simulink model "allmodes"  (Simulink 7.4)
settings: Solver=ode23tb  StartTime=0.0  StopTime=inf  MaxStep=1e-4  RelTol=1e-4
undefined symbols (not defined in the file): Ion, Lithium
libraries: powerlib x185, electricdrivelib x21, powerlib_extras x19, simulink x5
(part 6 of 7)

== system allmodes/battery controller /v16/Subsystem ==
  In1 : Inport
  Enable : EnablePort
  Constant2 : Constant  Value=0  OutDataType=fixdt(1, 16)  OutScaling=2^0
  Data Type Conversion2 : DataTypeConversion  OutDataType=fixdt(1, 16)  OutScaling=2^0
  Data Type Conversion3 : DataTypeConversion  OutDataType=fixdt(1, 16)  OutScaling=2^0
  Gain1 : Gain  Gain=-1  ParameterDataType=fixdt(1, 16)  ParameterScaling=2^0  OutDataType=fixdt(1, 16)  OutScaling=2^0
  Relational Operator2 : RelationalOperator  Operator=>  LogicOutDataTypeMode=boolean  LogicDataType=fixdt(0, 8)  OutDataTypeStr=boolean
  Relational Operator3 : RelationalOperator  Operator=>  LogicOutDataTypeMode=boolean  LogicDataType=fixdt(0, 8)  OutDataTypeStr=boolean
  Switch1 : Switch  OutDataType=fixdt(1, 16)  OutScaling=2^0
  Switch2 : Switch  Criteria=u2 > Threshold  OutDataType=fixdt(1, 16)  OutScaling=2^0
  sawtooth generator : Subsystem  mask{fsw=5e3, vc=1}
      mask prompts: fsw "switching frequency"; vc "magnitude"
  Out1 : Outport
  Out2 : Outport  Port=2
  wires:
  Switch1/1 -> Out2/1
  Switch2/1 -> Out1/1
  In1/1 -> Relational Operator2/1, Switch2/2, Switch1/2, Gain1/1
  Relational Operator3/1 -> Data Type Conversion2/1
  Relational Operator2/1 -> Data Type Conversion3/1
  Data Type Conversion3/1 -> Switch2/1
  Constant2/1 -> Switch2/3, Switch1/1
  Data Type Conversion2/1 -> Switch1/3
  sawtooth generator/1(saw) -> Relational Operator3/2, Relational Operator2/2
  Gain1/1 -> Relational Operator3/1

== system allmodes/battery controller /v16/Subsystem1 ==
  In1 : Inport
  Integrator : Integrator
  ain9 : Gain  Gain=5  ParameterDataType=fixdt(1, 16)  ParameterScaling=2^0  OutDataType=fixdt(1, 16)  OutScaling=2^0
  Out1 : Outport
  wires:
  In1/1 -> ain9/1
  Integrator/1 -> Out1/1
  ain9/1 -> Integrator/1

== system allmodes/battery controller /v16/Subsystem2 ==
  In1 : Inport
  Integrator : Integrator
  ain9 : Gain  Gain=5  ParameterDataType=fixdt(1, 16)  ParameterScaling=2^0  OutDataType=fixdt(1, 16)  OutScaling=2^0
  Out1 : Outport
  wires:
  ain9/1 -> Integrator/1
  Integrator/1 -> Out1/1
  In1/1 -> ain9/1

== system allmodes/battery controller /v16/Subsystem3 ==
  In1 : Inport
  Integrator : Integrator
  ain9 : Gain  Gain=5  ParameterDataType=fixdt(1, 16)  ParameterScaling=2^0  OutDataType=fixdt(1, 16)  OutScaling=2^0
  Out1 : Outport
  wires:
  In1/1 -> ain9/1
  Integrator/1 -> Out1/1
  ain9/1 -> Integrator/1

== system allmodes/battery controller /v17/Subsystem ==
  In1 : Inport
  Enable : EnablePort
  Constant2 : Constant  Value=0  OutDataType=fixdt(1, 16)  OutScaling=2^0
  Data Type Conversion2 : DataTypeConversion  OutDataType=fixdt(1, 16)  OutScaling=2^0
  Data Type Conversion3 : DataTypeConversion  OutDataType=fixdt(1, 16)  OutScaling=2^0
  Gain1 : Gain  Gain=-1  ParameterDataType=fixdt(1, 16)  ParameterScaling=2^0  OutDataType=fixdt(1, 16)  OutScaling=2^0
  Relational Operator2 : RelationalOperator  Operator=>  LogicOutDataTypeMode=boolean  LogicDataType=fixdt(0, 8)  OutDataTypeStr=boolean
  Relational Operator3 : RelationalOperator  Operator=>  LogicOutDataTypeMode=boolean  LogicDataType=fixdt(0, 8)  OutDataTypeStr=boolean
  Switch1 : Switch  OutDataType=fixdt(1, 16)  OutScaling=2^0
  Switch2 : Switch  Criteria=u2 > Threshold  OutDataType=fixdt(1, 16)  OutScaling=2^0
  sawtooth generator : Subsystem  mask{fsw=5e3, vc=1}
      mask prompts: fsw "switching frequency"; vc "magnitude"
  Out1 : Outport
  Out2 : Outport  Port=2
  wires:
  Switch1/1 -> Out2/1
  Switch2/1 -> Out1/1
  In1/1 -> Relational Operator2/1, Switch2/2, Switch1/2, Gain1/1
  Relational Operator3/1 -> Data Type Conversion2/1
  Relational Operator2/1 -> Data Type Conversion3/1
  Data Type Conversion3/1 -> Switch2/1
  Constant2/1 -> Switch2/3, Switch1/1
  Data Type Conversion2/1 -> Switch1/3
  sawtooth generator/1(saw) -> Relational Operator3/2, Relational Operator2/2
  Gain1/1 -> Relational Operator3/1

== system allmodes/battery controller /v17/Subsystem1 ==
  In1 : Inport
  Integrator : Integrator
  ain9 : Gain  Gain=5  ParameterDataType=fixdt(1, 16)  ParameterScaling=2^0  OutDataType=fixdt(1, 16)  OutScaling=2^0
  Out1 : Outport
  wires:
  In1/1 -> ain9/1
  Integrator/1 -> Out1/1
  ain9/1 -> Integrator/1

== system allmodes/battery controller /v17/Subsystem2 ==
  In1 : Inport
  Integrator : Integrator
  ain9 : Gain  Gain=5  ParameterDataType=fixdt(1, 16)  ParameterScaling=2^0  OutDataType=fixdt(1, 16)  OutScaling=2^0
  Out1 : Outport
  wires:
  ain9/1 -> Integrator/1
  Integrator/1 -> Out1/1
  In1/1 -> ain9/1

== system allmodes/battery controller /v17/Subsystem3 ==
  In1 : Inport
  Integrator : Integrator
  ain9 : Gain  Gain=5  ParameterDataType=fixdt(1, 16)  ParameterScaling=2^0  OutDataType=fixdt(1, 16)  OutScaling=2^0
  Out1 : Outport
  wires:
  In1/1 -> ain9/1
  Integrator/1 -> Out1/1
  ain9/1 -> Integrator/1

== system allmodes/battery controller /v18/Subsystem ==
  In1 : Inport
  Enable : EnablePort
  Constant2 : Constant  Value=0  OutDataType=fixdt(1, 16)  OutScaling=2^0
  Data Type Conversion2 : DataTypeConversion  OutDataType=fixdt(1, 16)  OutScaling=2^0
  Data Type Conversion3 : DataTypeConversion  OutDataType=fixdt(1, 16)  OutScaling=2^0
  Gain1 : Gain  Gain=-1  ParameterDataType=fixdt(1, 16)  ParameterScaling=2^0  OutDataType=fixdt(1, 16)  OutScaling=2^0
  Relational Operator2 : RelationalOperator  Operator=>  LogicOutDataTypeMode=boolean  LogicDataType=fixdt(0, 8)  OutDataTypeStr=boolean
  Relational Operator3 : RelationalOperator  Operator=>  LogicOutDataTypeMode=boolean  LogicDataType=fixdt(0, 8)  OutDataTypeStr=boolean
  Switch1 : Switch  OutDataType=fixdt(1, 16)  OutScaling=2^0
  Switch2 : Switch  Criteria=u2 > Threshold  OutDataType=fixdt(1, 16)  OutScaling=2^0
  sawtooth generator : Subsystem  mask{fsw=5e3, vc=1}
      mask prompts: fsw "switching frequency"; vc "magnitude"
  Out1 : Outport
  Out2 : Outport  Port=2
  wires:
  Switch1/1 -> Out2/1
  Switch2/1 -> Out1/1
  In1/1 -> Relational Operator2/1, Switch2/2, Switch1/2, Gain1/1
  Relational Operator3/1 -> Data Type Conversion2/1
  Relational Operator2/1 -> Data Type Conversion3/1
  Data Type Conversion3/1 -> Switch2/1
  Constant2/1 -> Switch2/3, Switch1/1
  Data Type Conversion2/1 -> Switch1/3
  sawtooth generator/1(saw) -> Relational Operator3/2, Relational Operator2/2
  Gain1/1 -> Relational Operator3/1

== system allmodes/battery controller /v18/Subsystem1 ==
  In1 : Inport
  Integrator : Integrator
  ain9 : Gain  Gain=5  ParameterDataType=fixdt(1, 16)  ParameterScaling=2^0  OutDataType=fixdt(1, 16)  OutScaling=2^0
  Out1 : Outport
  wires:
  In1/1 -> ain9/1
  Integrator/1 -> Out1/1
  ain9/1 -> Integrator/1

== system allmodes/battery controller /v18/Subsystem2 ==
  In1 : Inport
  Integrator : Integrator
  ain9 : Gain  Gain=5  ParameterDataType=fixdt(1, 16)  ParameterScaling=2^0  OutDataType=fixdt(1, 16)  OutScaling=2^0
  Out1 : Outport
  wires:
  ain9/1 -> Integrator/1
  Integrator/1 -> Out1/1
  In1/1 -> ain9/1

== system allmodes/battery controller /v18/Subsystem3 ==
  In1 : Inport
  Integrator : Integrator
  ain9 : Gain  Gain=5  ParameterDataType=fixdt(1, 16)  ParameterScaling=2^0  OutDataType=fixdt(1, 16)  OutScaling=2^0
  Out1 : Outport
  wires:
  In1/1 -> ain9/1
  Integrator/1 -> Out1/1
  ain9/1 -> Integrator/1

== system allmodes/battery controller /v19/Subsystem ==
  In1 : Inport
  Enable : EnablePort
  Constant2 : Constant  Value=0  OutDataType=fixdt(1, 16)  OutScaling=2^0
  Data Type Conversion2 : DataTypeConversion  OutDataType=fixdt(1, 16)  OutScaling=2^0
  Data Type Conversion3 : DataTypeConversion  OutDataType=fixdt(1, 16)  OutScaling=2^0
  Gain1 : Gain  Gain=-1  ParameterDataType=fixdt(1, 16)  ParameterScaling=2^0  OutDataType=fixdt(1, 16)  OutScaling=2^0
  Relational Operator2 : RelationalOperator  Operator=>  LogicOutDataTypeMode=boolean  LogicDataType=fixdt(0, 8)  OutDataTypeStr=boolean
  Relational Operator3 : RelationalOperator  Operator=>  LogicOutDataTypeMode=boolean  LogicDataType=fixdt(0, 8)  OutDataTypeStr=boolean
  Switch1 : Switch  OutDataType=fixdt(1, 16)  OutScaling=2^0
  Switch2 : Switch  Criteria=u2 > Threshold  OutDataType=fixdt(1, 16)  OutScaling=2^0
  sawtooth generator : Subsystem  mask{fsw=5e3, vc=1}
      mask prompts: fsw "switching frequency"; vc "magnitude"
  Out1 : Outport
  Out2 : Outport  Port=2
  wires:
  Switch1/1 -> Out2/1
  Switch2/1 -> Out1/1
  In1/1 -> Relational Operator2/1, Switch2/2, Switch1/2, Gain1/1
  Relational Operator3/1 -> Data Type Conversion2/1
  Relational Operator2/1 -> Data Type Conversion3/1
  Data Type Conversion3/1 -> Switch2/1
  Constant2/1 -> Switch2/3, Switch1/1
  Data Type Conversion2/1 -> Switch1/3
  sawtooth generator/1(saw) -> Relational Operator3/2, Relational Operator2/2
  Gain1/1 -> Relational Operator3/1

== system allmodes/battery controller /v19/Subsystem1 ==
  In1 : Inport
  Integrator : Integrator
  ain9 : Gain  Gain=5  ParameterDataType=fixdt(1, 16)  ParameterScaling=2^0  OutDataType=fixdt(1, 16)  OutScaling=2^0
  Out1 : Outport
  wires:
  In1/1 -> ain9/1
  Integrator/1 -> Out1/1
  ain9/1 -> Integrator/1

== system allmodes/battery controller /v19/Subsystem2 ==
  In1 : Inport
  Integrator : Integrator
  ain9 : Gain  Gain=5  ParameterDataType=fixdt(1, 16)  ParameterScaling=2^0  OutDataType=fixdt(1, 16)  OutScaling=2^0
  Out1 : Outport
  wires:
  ain9/1 -> Integrator/1
  Integrator/1 -> Out1/1
  In1/1 -> ain9/1

== system allmodes/battery controller /v19/Subsystem3 ==
  In1 : Inport
  Integrator : Integrator
  ain9 : Gain  Gain=5  ParameterDataType=fixdt(1, 16)  ParameterScaling=2^0  OutDataType=fixdt(1, 16)  OutScaling=2^0
  Out1 : Outport
  wires:
  In1/1 -> ain9/1
  Integrator/1 -> Out1/1
  ain9/1 -> Integrator/1

== system allmodes/battery controller /v2/Subsystem ==
  In1 : Inport
  Enable : EnablePort
  Constant2 : Constant  Value=0  OutDataType=fixdt(1, 16)  OutScaling=2^0
  Data Type Conversion2 : DataTypeConversion  OutDataType=fixdt(1, 16)  OutScaling=2^0
  Data Type Conversion3 : DataTypeConversion  OutDataType=fixdt(1, 16)  OutScaling=2^0
  Gain1 : Gain  Gain=-1  ParameterDataType=fixdt(1, 16)  ParameterScaling=2^0  OutDataType=fixdt(1, 16)  OutScaling=2^0
  Relational Operator2 : RelationalOperator  Operator=>  LogicOutDataTypeMode=boolean  LogicDataType=fixdt(0, 8)  OutDataTypeStr=boolean
  Relational Operator3 : RelationalOperator  Operator=>  LogicOutDataTypeMode=boolean  LogicDataType=fixdt(0, 8)  OutDataTypeStr=boolean
  Switch1 : Switch  OutDataType=fixdt(1, 16)  OutScaling=2^0
  Switch2 : Switch  Criteria=u2 > Threshold  OutDataType=fixdt(1, 16)  OutScaling=2^0
  sawtooth generator : Subsystem  mask{fsw=5e3, vc=1}
      mask prompts: fsw "switching frequency"; vc "magnitude"
  Out1 : Outport
  Out2 : Outport  Port=2
  wires:
  Relational Operator3/1 -> Data Type Conversion2/1
  Relational Operator2/1 -> Data Type Conversion3/1
  Data Type Conversion3/1 -> Switch2/1
  Constant2/1 -> Switch2/3, Switch1/1
  Data Type Conversion2/1 -> Switch1/3
  sawtooth generator/1(saw) -> Relational Operator3/2, Relational Operator2/2
  Gain1/1 -> Relational Operator3/1
  In1/1 -> Relational Operator2/1, Switch2/2, Switch1/2, Gain1/1
  Switch2/1 -> Out1/1
  Switch1/1 -> Out2/1

== system allmodes/battery controller /v2/Subsystem1 ==
  In1 : Inport
  Integrator : Integrator
  ain9 : Gain  Gain=5  ParameterDataType=fixdt(1, 16)  ParameterScaling=2^0  OutDataType=fixdt(1, 16)  OutScaling=2^0
  Out1 : Outport
  wires:
  In1/1 -> ain9/1
  Integrator/1 -> Out1/1
  ain9/1 -> Integrator/1

== system allmodes/battery controller /v2/Subsystem2 ==
  In1 : Inport
  Integrator : Integrator
  ain9 : Gain  Gain=5  ParameterDataType=fixdt(1, 16)  ParameterScaling=2^0  OutDataType=fixdt(1, 16)  OutScaling=2^0
  Out1 : Outport
  wires:
  ain9/1 -> Integrator/1
  Integrator/1 -> Out1/1
  In1/1 -> ain9/1

== system allmodes/battery controller /v2/Subsystem3 ==
  In1 : Inport
  Integrator : Integrator
  ain9 : Gain  Gain=5  ParameterDataType=fixdt(1, 16)  ParameterScaling=2^0  OutDataType=fixdt(1, 16)  OutScaling=2^0
  Out1 : Outport
  wires:
  In1/1 -> ain9/1
  Integrator/1 -> Out1/1
  ain9/1 -> Integrator/1

== system allmodes/battery controller /v20/Subsystem ==
  In1 : Inport
  Enable : EnablePort
  Constant2 : Constant  Value=0  OutDataType=fixdt(1, 16)  OutScaling=2^0
  Data Type Conversion2 : DataTypeConversion  OutDataType=fixdt(1, 16)  OutScaling=2^0
  Data Type Conversion3 : DataTypeConversion  OutDataType=fixdt(1, 16)  OutScaling=2^0
  Gain1 : Gain  Gain=-1  ParameterDataType=fixdt(1, 16)  ParameterScaling=2^0  OutDataType=fixdt(1, 16)  OutScaling=2^0
  Relational Operator2 : RelationalOperator  Operator=>  LogicOutDataTypeMode=boolean  LogicDataType=fixdt(0, 8)  OutDataTypeStr=boolean
  Relational Operator3 : RelationalOperator  Operator=>  LogicOutDataTypeMode=boolean  LogicDataType=fixdt(0, 8)  OutDataTypeStr=boolean
  Switch1 : Switch  OutDataType=fixdt(1, 16)  OutScaling=2^0
  Switch2 : Switch  Criteria=u2 > Threshold  OutDataType=fixdt(1, 16)  OutScaling=2^0
  sawtooth generator : Subsystem  mask{fsw=5e3, vc=1}
      mask prompts: fsw "switching frequency"; vc "magnitude"
  Out1 : Outport
  Out2 : Outport  Port=2
  wires:
  Switch1/1 -> Out2/1
  Switch2/1 -> Out1/1
  In1/1 -> Gain1/1, Switch1/2, Switch2/2, Relational Operator2/1
  Gain1/1 -> Relational Operator3/1
  sawtooth generator/1(saw) -> Relational Operator2/2, Relational Operator3/2
  Data Type Conversion2/1 -> Switch1/3
  Constant2/1 -> Switch1/1, Switch2/3
  Data Type Conversion3/1 -> Switch2/1
  Relational Operator2/1 -> Data Type Conversion3/1
  Relational Operator3/1 -> Data Type Conversion2/1

== system allmodes/battery controller /v20/Subsystem1 ==
  In1 : Inport
  Integrator : Integrator
  ain9 : Gain  Gain=5  ParameterDataType=fixdt(1, 16)  ParameterScaling=2^0  OutDataType=fixdt(1, 16)  OutScaling=2^0
  Out1 : Outport
  wires:
  ain9/1 -> Integrator/1
  Integrator/1 -> Out1/1
  In1/1 -> ain9/1

== system allmodes/battery controller /v20/Subsystem2 ==
  In1 : Inport
  Integrator : Integrator
  ain9 : Gain  Gain=5  ParameterDataType=fixdt(1, 16)  ParameterScaling=2^0  OutDataType=fixdt(1, 16)  OutScaling=2^0
  Out1 : Outport
  wires:
  In1/1 -> ain9/1
  Integrator/1 -> Out1/1
  ain9/1 -> Integrator/1

== system allmodes/battery controller /v20/Subsystem3 ==
  In1 : Inport
  Integrator : Integrator
  ain9 : Gain  Gain=5  ParameterDataType=fixdt(1, 16)  ParameterScaling=2^0  OutDataType=fixdt(1, 16)  OutScaling=2^0
  Out1 : Outport
  wires:
  ain9/1 -> Integrator/1
  Integrator/1 -> Out1/1
  In1/1 -> ain9/1

== system allmodes/battery controller /v3/Subsystem ==
  In1 : Inport
  Enable : EnablePort
  Constant2 : Constant  Value=0  OutDataType=fixdt(1, 16)  OutScaling=2^0
  Data Type Conversion2 : DataTypeConversion  OutDataType=fixdt(1, 16)  OutScaling=2^0
  Data Type Conversion3 : DataTypeConversion  OutDataType=fixdt(1, 16)  OutScaling=2^0
  Gain1 : Gain  Gain=-1  ParameterDataType=fixdt(1, 16)  ParameterScaling=2^0  OutDataType=fixdt(1, 16)  OutScaling=2^0
  Relational Operator2 : RelationalOperator  Operator=>  LogicOutDataTypeMode=boolean  LogicDataType=fixdt(0, 8)  OutDataTypeStr=boolean
  Relational Operator3 : RelationalOperator  Operator=>  LogicOutDataTypeMode=boolean  LogicDataType=fixdt(0, 8)  OutDataTypeStr=boolean
  Switch1 : Switch  OutDataType=fixdt(1, 16)  OutScaling=2^0
  Switch2 : Switch  Criteria=u2 > Threshold  OutDataType=fixdt(1, 16)  OutScaling=2^0
  sawtooth generator : Subsystem  mask{fsw=5e3, vc=1}
      mask prompts: fsw "switching frequency"; vc "magnitude"
  Out1 : Outport
  Out2 : Outport  Port=2
  wires:
  Switch1/1 -> Out2/1
  Switch2/1 -> Out1/1
  In1/1 -> Gain1/1, Switch1/2, Switch2/2, Relational Operator2/1
  Gain1/1 -> Relational Operator3/1
  sawtooth generator/1(saw) -> Relational Operator2/2, Relational Operator3/2
  Data Type Conversion2/1 -> Switch1/3
  Constant2/1 -> Switch1/1, Switch2/3
  Data Type Conversion3/1 -> Switch2/1
  Relational Operator2/1 -> Data Type Conversion3/1
  Relational Operator3/1 -> Data Type Conversion2/1

== system allmodes/battery controller /v3/Subsystem1 ==
  In1 : Inport
  Integrator : Integrator
  ain9 : Gain  Gain=5  ParameterDataType=fixdt(1, 16)  ParameterScaling=2^0  OutDataType=fixdt(1, 16)  OutScaling=2^0
  Out1 : Outport
  wires:
  ain9/1 -> Integrator/1
  Integrator/1 -> Out1/1
  In1/1 -> ain9/1

== system allmodes/battery controller /v3/Subsystem2 ==
  In1 : Inport
  Integrator : Integrator
  ain9 : Gain  Gain=5  ParameterDataType=fixdt(1, 16)  ParameterScaling=2^0  OutDataType=fixdt(1, 16)  OutScaling=2^0
  Out1 : Outport
  wires:
  In1/1 -> ain9/1
  Integrator/1 -> Out1/1
  ain9/1 -> Integrator/1

== system allmodes/battery controller /v3/Subsystem3 ==
  In1 : Inport
  Integrator : Integrator
  ain9 : Gain  Gain=5  ParameterDataType=fixdt(1, 16)  ParameterScaling=2^0  OutDataType=fixdt(1, 16)  OutScaling=2^0
  Out1 : Outport
  wires:
  ain9/1 -> Integrator/1
  Integrator/1 -> Out1/1
  In1/1 -> ain9/1

== system allmodes/battery controller /v4/Subsystem ==
  In1 : Inport
  Enable : EnablePort
  Constant2 : Constant  Value=0  OutDataType=fixdt(1, 16)  OutScaling=2^0
  Data Type Conversion2 : DataTypeConversion  OutDataType=fixdt(1, 16)  OutScaling=2^0
  Data Type Conversion3 : DataTypeConversion  OutDataType=fixdt(1, 16)  OutScaling=2^0
  Gain1 : Gain  Gain=-1  ParameterDataType=fixdt(1, 16)  ParameterScaling=2^0  OutDataType=fixdt(1, 16)  OutScaling=2^0
  Relational Operator2 : RelationalOperator  Operator=>  LogicOutDataTypeMode=boolean  LogicDataType=fixdt(0, 8)  OutDataTypeStr=boolean
  Relational Operator3 : RelationalOperator  Operator=>  LogicOutDataTypeMode=boolean  LogicDataType=fixdt(0, 8)  OutDataTypeStr=boolean
  Switch1 : Switch  OutDataType=fixdt(1, 16)  OutScaling=2^0
  Switch2 : Switch  Criteria=u2 > Threshold  OutDataType=fixdt(1, 16)  OutScaling=2^0
  sawtooth generator : Subsystem  mask{fsw=5e3, vc=1}
      mask prompts: fsw "switching frequency"; vc "magnitude"
  Out1 : Outport
  Out2 : Outport  Port=2
  wires:
  Relational Operator3/1 -> Data Type Conversion2/1
  Relational Operator2/1 -> Data Type Conversion3/1
  Data Type Conversion3/1 -> Switch2/1
  Constant2/1 -> Switch2/3, Switch1/1
  Data Type Conversion2/1 -> Switch1/3
  sawtooth generator/1(saw) -> Relational Operator3/2, Relational Operator2/2
  Gain1/1 -> Relational Operator3/1
  In1/1 -> Relational Operator2/1, Switch2/2, Switch1/2, Gain1/1
  Switch2/1 -> Out1/1
  Switch1/1 -> Out2/1

== system allmodes/battery controller /v4/Subsystem1 ==
  In1 : Inport
  Integrator : Integrator
  ain9 : Gain  Gain=5  ParameterDataType=fixdt(1, 16)  ParameterScaling=2^0  OutDataType=fixdt(1, 16)  OutScaling=2^0
  Out1 : Outport
  wires:
  In1/1 -> ain9/1
  Integrator/1 -> Out1/1
  ain9/1 -> Integrator/1

== system allmodes/battery controller /v4/Subsystem2 ==
  In1 : Inport
  Integrator : Integrator
  ain9 : Gain  Gain=5  ParameterDataType=fixdt(1, 16)  ParameterScaling=2^0  OutDataType=fixdt(1, 16)  OutScaling=2^0
  Out1 : Outport
  wires:
  ain9/1 -> Integrator/1
  Integrator/1 -> Out1/1
  In1/1 -> ain9/1

== system allmodes/battery controller /v4/Subsystem3 ==
  In1 : Inport
  Integrator : Integrator
  ain9 : Gain  Gain=5  ParameterDataType=fixdt(1, 16)  ParameterScaling=2^0  OutDataType=fixdt(1, 16)  OutScaling=2^0
  Out1 : Outport
  wires:
  In1/1 -> ain9/1
  Integrator/1 -> Out1/1
  ain9/1 -> Integrator/1

== system allmodes/battery controller /v5/Subsystem ==
  In1 : Inport
  Enable : EnablePort
  Constant2 : Constant  Value=0  OutDataType=fixdt(1, 16)  OutScaling=2^0
  Data Type Conversion2 : DataTypeConversion  OutDataType=fixdt(1, 16)  OutScaling=2^0
  Data Type Conversion3 : DataTypeConversion  OutDataType=fixdt(1, 16)  OutScaling=2^0
  Gain1 : Gain  Gain=-1  ParameterDataType=fixdt(1, 16)  ParameterScaling=2^0  OutDataType=fixdt(1, 16)  OutScaling=2^0
  Relational Operator2 : RelationalOperator  Operator=>  LogicOutDataTypeMode=boolean  LogicDataType=fixdt(0, 8)  OutDataTypeStr=boolean
  Relational Operator3 : RelationalOperator  Operator=>  LogicOutDataTypeMode=boolean  LogicDataType=fixdt(0, 8)  OutDataTypeStr=boolean
  Switch1 : Switch  OutDataType=fixdt(1, 16)  OutScaling=2^0
  Switch2 : Switch  Criteria=u2 > Threshold  OutDataType=fixdt(1, 16)  OutScaling=2^0
  sawtooth generator : Subsystem  mask{fsw=5e3, vc=1}
      mask prompts: fsw "switching frequency"; vc "magnitude"
  Out1 : Outport
  Out2 : Outport  Port=2
  wires:
  Switch1/1 -> Out2/1
  Switch2/1 -> Out1/1
  In1/1 -> Gain1/1, Switch1/2, Switch2/2, Relational Operator2/1
  Gain1/1 -> Relational Operator3/1
  sawtooth generator/1(saw) -> Relational Operator2/2, Relational Operator3/2
  Data Type Conversion2/1 -> Switch1/3
  Constant2/1 -> Switch1/1, Switch2/3
  Data Type Conversion3/1 -> Switch2/1
  Relational Operator2/1 -> Data Type Conversion3/1
  Relational Operator3/1 -> Data Type Conversion2/1

== system allmodes/battery controller /v5/Subsystem1 ==
  In1 : Inport
  Integrator : Integrator
  ain9 : Gain  Gain=5  ParameterDataType=fixdt(1, 16)  ParameterScaling=2^0  OutDataType=fixdt(1, 16)  OutScaling=2^0
  Out1 : Outport
  wires:
  ain9/1 -> Integrator/1
  Integrator/1 -> Out1/1
  In1/1 -> ain9/1

== system allmodes/battery controller /v5/Subsystem2 ==
  In1 : Inport
  Integrator : Integrator
  ain9 : Gain  Gain=5  ParameterDataType=fixdt(1, 16)  ParameterScaling=2^0  OutDataType=fixdt(1, 16)  OutScaling=2^0
  Out1 : Outport
  wires:
  In1/1 -> ain9/1
  Integrator/1 -> Out1/1
  ain9/1 -> Integrator/1

== system allmodes/battery controller /v5/Subsystem3 ==
  In1 : Inport
  Integrator : Integrator
  ain9 : Gain  Gain=5  ParameterDataType=fixdt(1, 16)  ParameterScaling=2^0  OutDataType=fixdt(1, 16)  OutScaling=2^0
  Out1 : Outport
  wires:
  ain9/1 -> Integrator/1
  Integrator/1 -> Out1/1
  In1/1 -> ain9/1

== system allmodes/battery controller /v6/Subsystem ==
  In1 : Inport
  Enable : EnablePort
  Constant2 : Constant  Value=0  OutDataType=fixdt(1, 16)  OutScaling=2^0
  Data Type Conversion2 : DataTypeConversion  OutDataType=fixdt(1, 16)  OutScaling=2^0
  Data Type Conversion3 : DataTypeConversion  OutDataType=fixdt(1, 16)  OutScaling=2^0
  Gain1 : Gain  Gain=-1  ParameterDataType=fixdt(1, 16)  ParameterScaling=2^0  OutDataType=fixdt(1, 16)  OutScaling=2^0
  Relational Operator2 : RelationalOperator  Operator=>  LogicOutDataTypeMode=boolean  LogicDataType=fixdt(0, 8)  OutDataTypeStr=boolean
  Relational Operator3 : RelationalOperator  Operator=>  LogicOutDataTypeMode=boolean  LogicDataType=fixdt(0, 8)  OutDataTypeStr=boolean
  Switch1 : Switch  OutDataType=fixdt(1, 16)  OutScaling=2^0
  Switch2 : Switch  Criteria=u2 > Threshold  OutDataType=fixdt(1, 16)  OutScaling=2^0
  sawtooth generator : Subsystem  mask{fsw=5e3, vc=1}
      mask prompts: fsw "switching frequency"; vc "magnitude"
  Out1 : Outport
  Out2 : Outport  Port=2
  wires:
  Relational Operator3/1 -> Data Type Conversion2/1
  Relational Operator2/1 -> Data Type Conversion3/1
  Data Type Conversion3/1 -> Switch2/1
  Constant2/1 -> Switch2/3, Switch1/1
  Data Type Conversion2/1 -> Switch1/3
  sawtooth generator/1(saw) -> Relational Operator3/2, Relational Operator2/2
  Gain1/1 -> Relational Operator3/1
  In1/1 -> Relational Operator2/1, Switch2/2, Switch1/2, Gain1/1
  Switch2/1 -> Out1/1
  Switch1/1 -> Out2/1

== system allmodes/battery controller /v6/Subsystem1 ==
  In1 : Inport
  Integrator : Integrator
  ain9 : Gain  Gain=5  ParameterDataType=fixdt(1, 16)  ParameterScaling=2^0  OutDataType=fixdt(1, 16)  OutScaling=2^0
  Out1 : Outport
  wires:
  In1/1 -> ain9/1
  Integrator/1 -> Out1/1
  ain9/1 -> Integrator/1

== system allmodes/battery controller /v6/Subsystem2 ==
  In1 : Inport
  Integrator : Integrator
  ain9 : Gain  Gain=5  ParameterDataType=fixdt(1, 16)  ParameterScaling=2^0  OutDataType=fixdt(1, 16)  OutScaling=2^0
  Out1 : Outport
  wires:
  ain9/1 -> Integrator/1
  Integrator/1 -> Out1/1
  In1/1 -> ain9/1

== system allmodes/battery controller /v6/Subsystem3 ==
  In1 : Inport
  Integrator : Integrator
  ain9 : Gain  Gain=5  ParameterDataType=fixdt(1, 16)  ParameterScaling=2^0  OutDataType=fixdt(1, 16)  OutScaling=2^0
  Out1 : Outport
  wires:
  In1/1 -> ain9/1
  Integrator/1 -> Out1/1
  ain9/1 -> Integrator/1

== system allmodes/battery controller /v7/Subsystem ==
  In1 : Inport
  Enable : EnablePort
  Constant2 : Constant  Value=0  OutDataType=fixdt(1, 16)  OutScaling=2^0
  Data Type Conversion2 : DataTypeConversion  OutDataType=fixdt(1, 16)  OutScaling=2^0
  Data Type Conversion3 : DataTypeConversion  OutDataType=fixdt(1, 16)  OutScaling=2^0
  Gain1 : Gain  Gain=-1  ParameterDataType=fixdt(1, 16)  ParameterScaling=2^0  OutDataType=fixdt(1, 16)  OutScaling=2^0
  Relational Operator2 : RelationalOperator  Operator=>  LogicOutDataTypeMode=boolean  LogicDataType=fixdt(0, 8)  OutDataTypeStr=boolean
  Relational Operator3 : RelationalOperator  Operator=>  LogicOutDataTypeMode=boolean  LogicDataType=fixdt(0, 8)  OutDataTypeStr=boolean
  Switch1 : Switch  OutDataType=fixdt(1, 16)  OutScaling=2^0
  Switch2 : Switch  Criteria=u2 > Threshold  OutDataType=fixdt(1, 16)  OutScaling=2^0
  sawtooth generator : Subsystem  mask{fsw=5e3, vc=1}
      mask prompts: fsw "switching frequency"; vc "magnitude"
  Out1 : Outport
  Out2 : Outport  Port=2
  wires:
  Switch1/1 -> Out2/1
  Switch2/1 -> Out1/1
  In1/1 -> Gain1/1, Switch1/2, Switch2/2, Relational Operator2/1
  Gain1/1 -> Relational Operator3/1
  sawtooth generator/1(saw) -> Relational Operator2/2, Relational Operator3/2
  Data Type Conversion2/1 -> Switch1/3
  Constant2/1 -> Switch1/1, Switch2/3
  Data Type Conversion3/1 -> Switch2/1
  Relational Operator2/1 -> Data Type Conversion3/1
  Relational Operator3/1 -> Data Type Conversion2/1

== system allmodes/battery controller /v7/Subsystem1 ==
  In1 : Inport
  Integrator : Integrator
  ain9 : Gain  Gain=5  ParameterDataType=fixdt(1, 16)  ParameterScaling=2^0  OutDataType=fixdt(1, 16)  OutScaling=2^0
  Out1 : Outport
  wires:
  ain9/1 -> Integrator/1
  Integrator/1 -> Out1/1
  In1/1 -> ain9/1

== system allmodes/battery controller /v7/Subsystem2 ==
  In1 : Inport
  Integrator : Integrator
  ain9 : Gain  Gain=5  ParameterDataType=fixdt(1, 16)  ParameterScaling=2^0  OutDataType=fixdt(1, 16)  OutScaling=2^0
  Out1 : Outport
  wires:
  In1/1 -> ain9/1
  Integrator/1 -> Out1/1
  ain9/1 -> Integrator/1

== system allmodes/battery controller /v7/Subsystem3 ==
  In1 : Inport
  Integrator : Integrator
  ain9 : Gain  Gain=5  ParameterDataType=fixdt(1, 16)  ParameterScaling=2^0  OutDataType=fixdt(1, 16)  OutScaling=2^0
  Out1 : Outport
  wires:
  ain9/1 -> Integrator/1
  Integrator/1 -> Out1/1
  In1/1 -> ain9/1

== system allmodes/battery controller /v8/Subsystem ==
  In1 : Inport
  Enable : EnablePort
  Constant2 : Constant  Value=0  OutDataType=fixdt(1, 16)  OutScaling=2^0
  Data Type Conversion2 : DataTypeConversion  OutDataType=fixdt(1, 16)  OutScaling=2^0
  Data Type Conversion3 : DataTypeConversion  OutDataType=fixdt(1, 16)  OutScaling=2^0
  Gain1 : Gain  Gain=-1  ParameterDataType=fixdt(1, 16)  ParameterScaling=2^0  OutDataType=fixdt(1, 16)  OutScaling=2^0
  Relational Operator2 : RelationalOperator  Operator=>  LogicOutDataTypeMode=boolean  LogicDataType=fixdt(0, 8)  OutDataTypeStr=boolean
  Relational Operator3 : RelationalOperator  Operator=>  LogicOutDataTypeMode=boolean  LogicDataType=fixdt(0, 8)  OutDataTypeStr=boolean
  Switch1 : Switch  OutDataType=fixdt(1, 16)  OutScaling=2^0
  Switch2 : Switch  Criteria=u2 > Threshold  OutDataType=fixdt(1, 16)  OutScaling=2^0
  sawtooth generator : Subsystem  mask{fsw=5e3, vc=1}
      mask prompts: fsw "switching frequency"; vc "magnitude"
  Out1 : Outport
  Out2 : Outport  Port=2
  wires:
  Relational Operator3/1 -> Data Type Conversion2/1
  Relational Operator2/1 -> Data Type Conversion3/1
  Data Type Conversion3/1 -> Switch2/1
  Constant2/1 -> Switch2/3, Switch1/1
  Data Type Conversion2/1 -> Switch1/3
  sawtooth generator/1(saw) -> Relational Operator3/2, Relational Operator2/2
  Gain1/1 -> Relational Operator3/1
  In1/1 -> Relational Operator2/1, Switch2/2, Switch1/2, Gain1/1
  Switch2/1 -> Out1/1
  Switch1/1 -> Out2/1

== system allmodes/battery controller /v8/Subsystem1 ==
  In1 : Inport
  Integrator : Integrator
  ain9 : Gain  Gain=5  ParameterDataType=fixdt(1, 16)  ParameterScaling=2^0  OutDataType=fixdt(1, 16)  OutScaling=2^0
  Out1 : Outport
  wires:
  In1/1 -> ain9/1
  Integrator/1 -> Out1/1
  ain9/1 -> Integrator/1

== system allmodes/battery controller /v8/Subsystem2 ==
  In1 : Inport
  Integrator : Integrator
  ain9 : Gain  Gain=5  ParameterDataType=fixdt(1, 16)  ParameterScaling=2^0  OutDataType=fixdt(1, 16)  OutScaling=2^0
  Out1 : Outport
  wires:
  ain9/1 -> Integrator/1
  Integrator/1 -> Out1/1
  In1/1 -> ain9/1

== system allmodes/battery controller /v8/Subsystem3 ==
  In1 : Inport
  Integrator : Integrator
  ain9 : Gain  Gain=5  ParameterDataType=fixdt(1, 16)  ParameterScaling=2^0  OutDataType=fixdt(1, 16)  OutScaling=2^0
  Out1 : Outport
  wires:
  In1/1 -> ain9/1
  Integrator/1 -> Out1/1
  ain9/1 -> Integrator/1

== system allmodes/battery controller /v9/Subsystem ==
  In1 : Inport
  Enable : EnablePort
  Constant2 : Constant  Value=0  OutDataType=fixdt(1, 16)  OutScaling=2^0
  Data Type Conversion2 : DataTypeConversion  OutDataType=fixdt(1, 16)  OutScaling=2^0
  Data Type Conversion3 : DataTypeConversion  OutDataType=fixdt(1, 16)  OutScaling=2^0
  Gain1 : Gain  Gain=-1  ParameterDataType=fixdt(1, 16)  ParameterScaling=2^0  OutDataType=fixdt(1, 16)  OutScaling=2^0
  Relational Operator2 : RelationalOperator  Operator=>  LogicOutDataTypeMode=boolean  LogicDataType=fixdt(0, 8)  OutDataTypeStr=boolean
  Relational Operator3 : RelationalOperator  Operator=>  LogicOutDataTypeMode=boolean  LogicDataType=fixdt(0, 8)  OutDataTypeStr=boolean
  Switch1 : Switch  OutDataType=fixdt(1, 16)  OutScaling=2^0
  Switch2 : Switch  Criteria=u2 > Threshold  OutDataType=fixdt(1, 16)  OutScaling=2^0
  sawtooth generator : Subsystem  mask{fsw=5e3, vc=1}
      mask prompts: fsw "switching frequency"; vc "magnitude"
  Out1 : Outport
  Out2 : Outport  Port=2
  wires:
  Switch1/1 -> Out2/1
  Switch2/1 -> Out1/1
  In1/1 -> Gain1/1, Switch1/2, Switch2/2, Relational Operator2/1
  Gain1/1 -> Relational Operator3/1
  sawtooth generator/1(saw) -> Relational Operator2/2, Relational Operator3/2
  Data Type Conversion2/1 -> Switch1/3
  Constant2/1 -> Switch1/1, Switch2/3
  Data Type Conversion3/1 -> Switch2/1
  Relational Operator2/1 -> Data Type Conversion3/1
  Relational Operator3/1 -> Data Type Conversion2/1

== system allmodes/battery controller /v9/Subsystem1 ==
  In1 : Inport
  Integrator : Integrator
  ain9 : Gain  Gain=5  ParameterDataType=fixdt(1, 16)  ParameterScaling=2^0  OutDataType=fixdt(1, 16)  OutScaling=2^0
  Out1 : Outport
  wires:
  ain9/1 -> Integrator/1
  Integrator/1 -> Out1/1
  In1/1 -> ain9/1

== system allmodes/battery controller /v9/Subsystem2 ==
  In1 : Inport
  Integrator : Integrator
  ain9 : Gain  Gain=5  ParameterDataType=fixdt(1, 16)  ParameterScaling=2^0  OutDataType=fixdt(1, 16)  OutScaling=2^0
  Out1 : Outport
  wires:
  In1/1 -> ain9/1
  Integrator/1 -> Out1/1
  ain9/1 -> Integrator/1

== system allmodes/battery controller /v9/Subsystem3 ==
  In1 : Inport
  Integrator : Integrator
  ain9 : Gain  Gain=5  ParameterDataType=fixdt(1, 16)  ParameterScaling=2^0  OutDataType=fixdt(1, 16)  OutScaling=2^0
  Out1 : Outport
  wires:
  ain9/1 -> Integrator/1
  Integrator/1 -> Out1/1
  In1/1 -> ain9/1

== system allmodes/vechicle units/vechicle-1/IGBT20 ==
  IGBT/Diode : powerlib/Power Electronics/IGBT//Diode  DialogController=POWERSYS.PowerSysDialog  SystemSampleTime=-1  Ron=1e-3  Rs=1e5  Cs=inf  Measurements=off
  collector : PMIOPort  Port=1  Side=Right
  emitter : PMIOPort  Port=2  Side=Right
  wires:
  [buckv1] -> IGBT/Diode/1
  connections:
  collector/RConn1 -- IGBT/Diode/LConn1
  emitter/RConn1 -- IGBT/Diode/RConn1

== system allmodes/vechicle units/vechicle-1/IGBT21 ==
  IGBT/Diode : powerlib/Power Electronics/IGBT//Diode  DialogController=POWERSYS.PowerSysDialog  SystemSampleTime=-1  Ron=1e-3  Rs=1e5  Cs=inf  Measurements=off
  collector : PMIOPort  Port=1  Side=Right
  emitter : PMIOPort  Port=2  Side=Right
  wires:
  [boostv1] -> IGBT/Diode/1
  connections:
  emitter/RConn1 -- IGBT/Diode/RConn1
  collector/RConn1 -- IGBT/Diode/LConn1

== system allmodes/vechicle units/vechicle-10/IGBT20 ==
  IGBT/Diode : powerlib/Power Electronics/IGBT//Diode  DialogController=POWERSYS.PowerSysDialog  SystemSampleTime=-1  Ron=1e-3  Rs=1e5  Cs=inf  Measurements=off
  collector : PMIOPort  Port=1  Side=Right
  emitter : PMIOPort  Port=2  Side=Right
  wires:
  [buckv10] -> IGBT/Diode/1
  connections:
  emitter/RConn1 -- IGBT/Diode/RConn1
  collector/RConn1 -- IGBT/Diode/LConn1

== system allmodes/vechicle units/vechicle-10/IGBT21 ==
  IGBT/Diode : powerlib/Power Electronics/IGBT//Diode  DialogController=POWERSYS.PowerSysDialog  SystemSampleTime=-1  Ron=1e-3  Rs=1e5  Cs=inf  Measurements=off
  collector : PMIOPort  Port=1  Side=Right
  emitter : PMIOPort  Port=2  Side=Right
  wires:
  [boostv10] -> IGBT/Diode/1
  connections:
  collector/RConn1 -- IGBT/Diode/LConn1
  emitter/RConn1 -- IGBT/Diode/RConn1

== system allmodes/vechicle units/vechicle-11/IGBT20 ==
  IGBT/Diode : powerlib/Power Electronics/IGBT//Diode  DialogController=POWERSYS.PowerSysDialog  SystemSampleTime=-1  Ron=1e-3  Rs=1e5  Cs=inf  Measurements=off
  collector : PMIOPort  Port=1  Side=Right
  emitter : PMIOPort  Port=2  Side=Right
  wires:
  [buckv11] -> IGBT/Diode/1
  connections:
  collector/RConn1 -- IGBT/Diode/LConn1
  emitter/RConn1 -- IGBT/Diode/RConn1

== system allmodes/vechicle units/vechicle-11/IGBT21 ==
  IGBT/Diode : powerlib/Power Electronics/IGBT//Diode  DialogController=POWERSYS.PowerSysDialog  SystemSampleTime=-1  Ron=1e-3  Rs=1e5  Cs=inf  Measurements=off
  collector : PMIOPort  Port=1  Side=Right
  emitter : PMIOPort  Port=2  Side=Right
  wires:
  [boostv11] -> IGBT/Diode/1
  connections:
  emitter/RConn1 -- IGBT/Diode/RConn1
  collector/RConn1 -- IGBT/Diode/LConn1

== system allmodes/vechicle units/vechicle-12/IGBT20 ==
  IGBT/Diode : powerlib/Power Electronics/IGBT//Diode  DialogController=POWERSYS.PowerSysDialog  SystemSampleTime=-1  Ron=1e-3  Rs=1e5  Cs=inf  Measurements=off
  collector : PMIOPort  Port=1  Side=Right
  emitter : PMIOPort  Port=2  Side=Right
  wires:
  [buckv12] -> IGBT/Diode/1
  connections:
  emitter/RConn1 -- IGBT/Diode/RConn1
  collector/RConn1 -- IGBT/Diode/LConn1

== system allmodes/vechicle units/vechicle-12/IGBT21 ==
  IGBT/Diode : powerlib/Power Electronics/IGBT//Diode  DialogController=POWERSYS.PowerSysDialog  SystemSampleTime=-1  Ron=1e-3  Rs=1e5  Cs=inf  Measurements=off
  collector : PMIOPort  Port=1  Side=Right
  emitter : PMIOPort  Port=2  Side=Right
  wires:
  [boostv12] -> IGBT/Diode/1
  connections:
  collector/RConn1 -- IGBT/Diode/LConn1
  emitter/RConn1 -- IGBT/Diode/RConn1

== system allmodes/vechicle units/vechicle-13/IGBT20 ==
  IGBT/Diode : powerlib/Power Electronics/IGBT//Diode  DialogController=POWERSYS.PowerSysDialog  SystemSampleTime=-1  Ron=1e-3  Rs=1e5  Cs=inf  Measurements=off
  collector : PMIOPort  Port=1  Side=Right
  emitter : PMIOPort  Port=2  Side=Right
  wires:
  [buckv13] -> IGBT/Diode/1
  connections:
  collector/RConn1 -- IGBT/Diode/LConn1
  emitter/RConn1 -- IGBT/Diode/RConn1

== system allmodes/vechicle units/vechicle-13/IGBT21 ==
  IGBT/Diode : powerlib/Power Electronics/IGBT//Diode  DialogController=POWERSYS.PowerSysDialog  SystemSampleTime=-1  Ron=1e-3  Rs=1e5  Cs=inf  Measurements=off
  collector : PMIOPort  Port=1  Side=Right
  emitter : PMIOPort  Port=2  Side=Right
  wires:
  [boostv13] -> IGBT/Diode/1
  connections:
  emitter/RConn1 -- IGBT/Diode/RConn1
  collector/RConn1 -- IGBT/Diode/LConn1

== system allmodes/vechicle units/vechicle-14/IGBT20 ==
  IGBT/Diode : powerlib/Power Electronics/IGBT//Diode  DialogController=POWERSYS.PowerSysDialog  SystemSampleTime=-1  Ron=1e-3  Rs=1e5  Cs=inf  Measurements=off
  collector : PMIOPort  Port=1  Side=Right
  emitter : PMIOPort  Port=2  Side=Right
  wires:
  [buckv14] -> IGBT/Diode/1
  connections:
  emitter/RConn1 -- IGBT/Diode/RConn1
  collector/RConn1 -- IGBT/Diode/LConn1

== system allmodes/vechicle units/vechicle-14/IGBT21 ==
  IGBT/Diode : powerlib/Power Electronics/IGBT//Diode  DialogController=POWERSYS.PowerSysDialog  SystemSampleTime=-1  Ron=1e-3  Rs=1e5  Cs=inf  Measurements=off
  collector : PMIOPort  Port=1  Side=Right
  emitter : PMIOPort  Port=2  Side=Right
  wires:
  [boostv14] -> IGBT/Diode/1
  connections:
  collector/RConn1 -- IGBT/Diode/LConn1
  emitter/RConn1 -- IGBT/Diode/RConn1

== system allmodes/vechicle units/vechicle-15/IGBT20 ==
  IGBT/Diode : powerlib/Power Electronics/IGBT//Diode  DialogController=POWERSYS.PowerSysDialog  SystemSampleTime=-1  Ron=1e-3  Rs=1e5  Cs=inf  Measurements=off
  collector : PMIOPort  Port=1  Side=Right
  emitter : PMIOPort  Port=2  Side=Right
  wires:
  [buckv15] -> IGBT/Diode/1
  connections:
  collector/RConn1 -- IGBT/Diode/LConn1
  emitter/RConn1 -- IGBT/Diode/RConn1

== system allmodes/vechicle units/vechicle-15/IGBT21 ==
  IGBT/Diode : powerlib/Power Electronics/IGBT//Diode  DialogController=POWERSYS.PowerSysDialog  SystemSampleTime=-1  Ron=1e-3  Rs=1e5  Cs=inf  Measurements=off
  collector : PMIOPort  Port=1  Side=Right
  emitter : PMIOPort  Port=2  Side=Right
  wires:
  [boostv15] -> IGBT/Diode/1
  connections:
  emitter/RConn1 -- IGBT/Diode/RConn1
  collector/RConn1 -- IGBT/Diode/LConn1

== system allmodes/vechicle units/vechicle-16/IGBT20 ==
  IGBT/Diode : powerlib/Power Electronics/IGBT//Diode  DialogController=POWERSYS.PowerSysDialog  SystemSampleTime=-1  Ron=1e-3  Rs=1e5  Cs=inf  Measurements=off
  collector : PMIOPort  Port=1  Side=Right
  emitter : PMIOPort  Port=2  Side=Right
  wires:
  [buckv16] -> IGBT/Diode/1
  connections:
  emitter/RConn1 -- IGBT/Diode/RConn1
  collector/RConn1 -- IGBT/Diode/LConn1

== system allmodes/vechicle units/vechicle-16/IGBT21 ==
  IGBT/Diode : powerlib/Power Electronics/IGBT//Diode  DialogController=POWERSYS.PowerSysDialog  SystemSampleTime=-1  Ron=1e-3  Rs=1e5  Cs=inf  Measurements=off
  collector : PMIOPort  Port=1  Side=Right
  emitter : PMIOPort  Port=2  Side=Right
  wires:
  [boostv16] -> IGBT/Diode/1
  connections:
  collector/RConn1 -- IGBT/Diode/LConn1
  emitter/RConn1 -- IGBT/Diode/RConn1

== system allmodes/vechicle units/vechicle-17/IGBT20 ==
  IGBT/Diode : powerlib/Power Electronics/IGBT//Diode  DialogController=POWERSYS.PowerSysDialog  SystemSampleTime=-1  Ron=1e-3  Rs=1e5  Cs=inf  Measurements=off
  collector : PMIOPort  Port=1  Side=Right
  emitter : PMIOPort  Port=2  Side=Right
  wires:
  [buckv17] -> IGBT/Diode/1
  connections:
  collector/RConn1 -- IGBT/Diode/LConn1
  emitter/RConn1 -- IGBT/Diode/RConn1

== system allmodes/vechicle units/vechicle-17/IGBT21 ==
  IGBT/Diode : powerlib/Power Electronics/IGBT//Diode  DialogController=POWERSYS.PowerSysDialog  SystemSampleTime=-1  Ron=1e-3  Rs=1e5  Cs=inf  Measurements=off
  collector : PMIOPort  Port=1  Side=Right
  emitter : PMIOPort  Port=2  Side=Right
  wires:
  [boostv17] -> IGBT/Diode/1
  connections:
  emitter/RConn1 -- IGBT/Diode/RConn1
  collector/RConn1 -- IGBT/Diode/LConn1

== system allmodes/vechicle units/vechicle-18/IGBT20 ==
  IGBT/Diode : powerlib/Power Electronics/IGBT//Diode  DialogController=POWERSYS.PowerSysDialog  SystemSampleTime=-1  Ron=1e-3  Rs=1e5  Cs=inf  Measurements=off
  collector : PMIOPort  Port=1  Side=Right
  emitter : PMIOPort  Port=2  Side=Right
  wires:
  [buckv18] -> IGBT/Diode/1
  connections:
  emitter/RConn1 -- IGBT/Diode/RConn1
  collector/RConn1 -- IGBT/Diode/LConn1

== system allmodes/vechicle units/vechicle-18/IGBT21 ==
  IGBT/Diode : powerlib/Power Electronics/IGBT//Diode  DialogController=POWERSYS.PowerSysDialog  SystemSampleTime=-1  Ron=1e-3  Rs=1e5  Cs=inf  Measurements=off
  collector : PMIOPort  Port=1  Side=Right
  emitter : PMIOPort  Port=2  Side=Right
  wires:
  [boostv18] -> IGBT/Diode/1
  connections:
  collector/RConn1 -- IGBT/Diode/LConn1
  emitter/RConn1 -- IGBT/Diode/RConn1

== system allmodes/vechicle units/vechicle-19/IGBT20 ==
  IGBT/Diode : powerlib/Power Electronics/IGBT//Diode  DialogController=POWERSYS.PowerSysDialog  SystemSampleTime=-1  Ron=1e-3  Rs=1e5  Cs=inf  Measurements=off
  collector : PMIOPort  Port=1  Side=Right
  emitter : PMIOPort  Port=2  Side=Right
  wires:
  [buckv19] -> IGBT/Diode/1
  connections:
  collector/RConn1 -- IGBT/Diode/LConn1
  emitter/RConn1 -- IGBT/Diode/RConn1

== system allmodes/vechicle units/vechicle-19/IGBT21 ==
  IGBT/Diode : powerlib/Power Electronics/IGBT//Diode  DialogController=POWERSYS.PowerSysDialog  SystemSampleTime=-1  Ron=1e-3  Rs=1e5  Cs=inf  Measurements=off
  collector : PMIOPort  Port=1  Side=Right
  emitter : PMIOPort  Port=2  Side=Right
  wires:
  [boostv19] -> IGBT/Diode/1
  connections:
  emitter/RConn1 -- IGBT/Diode/RConn1
  collector/RConn1 -- IGBT/Diode/LConn1

== system allmodes/vechicle units/vechicle-2/IGBT20 ==
  IGBT/Diode : powerlib/Power Electronics/IGBT//Diode  DialogController=POWERSYS.PowerSysDialog  SystemSampleTime=-1  Ron=1e-3  Rs=1e5  Cs=inf  Measurements=off
  collector : PMIOPort  Port=1  Side=Right
  emitter : PMIOPort  Port=2  Side=Right
  wires:
  [buckv2] -> IGBT/Diode/1
  connections:
  emitter/RConn1 -- IGBT/Diode/RConn1
  collector/RConn1 -- IGBT/Diode/LConn1

== system allmodes/vechicle units/vechicle-2/IGBT21 ==
  IGBT/Diode : powerlib/Power Electronics/IGBT//Diode  DialogController=POWERSYS.PowerSysDialog  SystemSampleTime=-1  Ron=1e-3  Rs=1e5  Cs=inf  Measurements=off
  collector : PMIOPort  Port=1  Side=Right
  emitter : PMIOPort  Port=2  Side=Right
  wires:
  [boostv2] -> IGBT/Diode/1
  connections:
  collector/RConn1 -- IGBT/Diode/LConn1
  emitter/RConn1 -- IGBT/Diode/RConn1

== system allmodes/vechicle units/vechicle-20/IGBT20 ==
  IGBT/Diode : powerlib/Power Electronics/IGBT//Diode  DialogController=POWERSYS.PowerSysDialog  SystemSampleTime=-1  Ron=1e-3  Rs=1e5  Cs=inf  Measurements=off
  collector : PMIOPort  Port=1  Side=Right
  emitter : PMIOPort  Port=2  Side=Right
  wires:
  [buckv20] -> IGBT/Diode/1
  connections:
  emitter/RConn1 -- IGBT/Diode/RConn1
  collector/RConn1 -- IGBT/Diode/LConn1

== system allmodes/vechicle units/vechicle-20/IGBT21 ==
  IGBT/Diode : powerlib/Power Electronics/IGBT//Diode  DialogController=POWERSYS.PowerSysDialog  SystemSampleTime=-1  Ron=1e-3  Rs=1e5  Cs=inf  Measurements=off
  collector : PMIOPort  Port=1  Side=Right
  emitter : PMIOPort  Port=2  Side=Right
  wires:
  [boostv20] -> IGBT/Diode/1
  connections:
  collector/RConn1 -- IGBT/Diode/LConn1
  emitter/RConn1 -- IGBT/Diode/RConn1

== system allmodes/vechicle units/vechicle-3/IGBT20 ==
  IGBT/Diode : powerlib/Power Electronics/IGBT//Diode  DialogController=POWERSYS.PowerSysDialog  SystemSampleTime=-1  Ron=1e-3  Rs=1e5  Cs=inf  Measurements=off
  collector : PMIOPort  Port=1  Side=Right
  emitter : PMIOPort  Port=2  Side=Right
  wires:
  [buckv3] -> IGBT/Diode/1
  connections:
  collector/RConn1 -- IGBT/Diode/LConn1
  emitter/RConn1 -- IGBT/Diode/RConn1

== system allmodes/vechicle units/vechicle-3/IGBT21 ==
  IGBT/Diode : powerlib/Power Electronics/IGBT//Diode  DialogController=POWERSYS.PowerSysDialog  SystemSampleTime=-1  Ron=1e-3  Rs=1e5  Cs=inf  Measurements=off
  collector : PMIOPort  Port=1  Side=Right
  emitter : PMIOPort  Port=2  Side=Right
  wires:
  [boostv3] -> IGBT/Diode/1
  connections:
  emitter/RConn1 -- IGBT/Diode/RConn1
  collector/RConn1 -- IGBT/Diode/LConn1

== system allmodes/vechicle units/vechicle-4/IGBT20 ==
  IGBT/Diode : powerlib/Power Electronics/IGBT//Diode  DialogController=POWERSYS.PowerSysDialog  SystemSampleTime=-1  Ron=1e-3  Rs=1e5  Cs=inf  Measurements=off
  collector : PMIOPort  Port=1  Side=Right
  emitter : PMIOPort  Port=2  Side=Right
  wires:
  [buckv4] -> IGBT/Diode/1
  connections:
  emitter/RConn1 -- IGBT/Diode/RConn1
  collector/RConn1 -- IGBT/Diode/LConn1

== system allmodes/vechicle units/vechicle-4/IGBT21 ==
  IGBT/Diode : powerlib/Power Electronics/IGBT//Diode  DialogController=POWERSYS.PowerSysDialog  SystemSampleTime=-1  Ron=1e-3  Rs=1e5  Cs=inf  Measurements=off
  collector : PMIOPort  Port=1  Side=Right
  emitter : PMIOPort  Port=2  Side=Right
  wires:
  [boostv4] -> IGBT/Diode/1
  connections:
  collector/RConn1 -- IGBT/Diode/LConn1
  emitter/RConn1 -- IGBT/Diode/RConn1

== system allmodes/vechicle units/vechicle-5/IGBT20 ==
  IGBT/Diode : powerlib/Power Electronics/IGBT//Diode  DialogController=POWERSYS.PowerSysDialog  SystemSampleTime=-1  Ron=1e-3  Rs=1e5  Cs=inf  Measurements=off
  collector : PMIOPort  Port=1  Side=Right
  emitter : PMIOPort  Port=2  Side=Right
  wires:
  [buckv5] -> IGBT/Diode/1
  connections:
  collector/RConn1 -- IGBT/Diode/LConn1
  emitter/RConn1 -- IGBT/Diode/RConn1

== system allmodes/vechicle units/vechicle-5/IGBT21 ==
  IGBT/Diode : powerlib/Power Electronics/IGBT//Diode  DialogController=POWERSYS.PowerSysDialog  SystemSampleTime=-1  Ron=1e-3  Rs=1e5  Cs=inf  Measurements=off
  collector : PMIOPort  Port=1  Side=Right
  emitter : PMIOPort  Port=2  Side=Right
  wires:
  [boostv5] -> IGBT/Diode/1
  connections:
  emitter/RConn1 -- IGBT/Diode/RConn1
  collector/RConn1 -- IGBT/Diode/LConn1

== system allmodes/vechicle units/vechicle-6/IGBT20 ==
  IGBT/Diode : powerlib/Power Electronics/IGBT//Diode  DialogController=POWERSYS.PowerSysDialog  SystemSampleTime=-1  Ron=1e-3  Rs=1e5  Cs=inf  Measurements=off
  collector : PMIOPort  Port=1  Side=Right
  emitter : PMIOPort  Port=2  Side=Right
  wires:
  [buckv6] -> IGBT/Diode/1
  connections:
  emitter/RConn1 -- IGBT/Diode/RConn1
  collector/RConn1 -- IGBT/Diode/LConn1

== system allmodes/vechicle units/vechicle-6/IGBT21 ==
  IGBT/Diode : powerlib/Power Electronics/IGBT//Diode  DialogController=POWERSYS.PowerSysDialog  SystemSampleTime=-1  Ron=1e-3  Rs=1e5  Cs=inf  Measurements=off
  collector : PMIOPort  Port=1  Side=Right
  emitter : PMIOPort  Port=2  Side=Right
  wires:
  [boostv6] -> IGBT/Diode/1
  connections:
  collector/RConn1 -- IGBT/Diode/LConn1
  emitter/RConn1 -- IGBT/Diode/RConn1

== system allmodes/vechicle units/vechicle-7/IGBT20 ==
  IGBT/Diode : powerlib/Power Electronics/IGBT//Diode  DialogController=POWERSYS.PowerSysDialog  SystemSampleTime=-1  Ron=1e-3  Rs=1e5  Cs=inf  Measurements=off
  collector : PMIOPort  Port=1  Side=Right
  emitter : PMIOPort  Port=2  Side=Right
  wires:
  [buckv7] -> IGBT/Diode/1
  connections:
  collector/RConn1 -- IGBT/Diode/LConn1
  emitter/RConn1 -- IGBT/Diode/RConn1

== system allmodes/vechicle units/vechicle-7/IGBT21 ==
  IGBT/Diode : powerlib/Power Electronics/IGBT//Diode  DialogController=POWERSYS.PowerSysDialog  SystemSampleTime=-1  Ron=1e-3  Rs=1e5  Cs=inf  Measurements=off
  collector : PMIOPort  Port=1  Side=Right
  emitter : PMIOPort  Port=2  Side=Right
  wires:
  [boostv7] -> IGBT/Diode/1
  connections:
  emitter/RConn1 -- IGBT/Diode/RConn1
  collector/RConn1 -- IGBT/Diode/LConn1

== system allmodes/vechicle units/vechicle-8/IGBT20 ==
  IGBT/Diode : powerlib/Power Electronics/IGBT//Diode  DialogController=POWERSYS.PowerSysDialog  SystemSampleTime=-1  Ron=1e-3  Rs=1e5  Cs=inf  Measurements=off
  collector : PMIOPort  Port=1  Side=Right
  emitter : PMIOPort  Port=2  Side=Right
  wires:
  [buckv8] -> IGBT/Diode/1
  connections:
  emitter/RConn1 -- IGBT/Diode/RConn1
  collector/RConn1 -- IGBT/Diode/LConn1

== system allmodes/vechicle units/vechicle-8/IGBT21 ==
  IGBT/Diode : powerlib/Power Electronics/IGBT//Diode  DialogController=POWERSYS.PowerSysDialog  SystemSampleTime=-1  Ron=1e-3  Rs=1e5  Cs=inf  Measurements=off
  collector : PMIOPort  Port=1  Side=Right
  emitter : PMIOPort  Port=2  Side=Right
  wires:
  [boostv8] -> IGBT/Diode/1
  connections:
  collector/RConn1 -- IGBT/Diode/LConn1
  emitter/RConn1 -- IGBT/Diode/RConn1

== system allmodes/vechicle units/vechicle-9/IGBT20 ==
  IGBT/Diode : powerlib/Power Electronics/IGBT//Diode  DialogController=POWERSYS.PowerSysDialog  SystemSampleTime=-1  Ron=1e-3  Rs=1e5  Cs=inf  Measurements=off
  collector : PMIOPort  Port=1  Side=Right
  emitter : PMIOPort  Port=2  Side=Right
  wires:
  [buckv9] -> IGBT/Diode/1
  connections:
  collector/RConn1 -- IGBT/Diode/LConn1
  emitter/RConn1 -- IGBT/Diode/RConn1

== system allmodes/vechicle units/vechicle-9/IGBT21 ==
  IGBT/Diode : powerlib/Power Electronics/IGBT//Diode  DialogController=POWERSYS.PowerSysDialog  SystemSampleTime=-1  Ron=1e-3  Rs=1e5  Cs=inf  Measurements=off
  collector : PMIOPort  Port=1  Side=Right
  emitter : PMIOPort  Port=2  Side=Right
  wires:
  [boostv9] -> IGBT/Diode/1
  connections:
  emitter/RConn1 -- IGBT/Diode/RConn1
  collector/RConn1 -- IGBT/Diode/LConn1

== system allmodes/battery controller /SUIM1/Subsystem/sawtooth generator ==
  Clock : Clock
      settings: DisableCoverage=on  Decimation=10
  Constant : Constant  DisableCoverage=on  Value=1/fsw  OutDataType=fixdt(1, 16)  OutScaling=2^0
  Divide : Product  Inputs=*/  OutDataType=fixdt(1, 16)  OutScaling=2^-10
  Gain : Gain  Gain=vc  ParameterDataType=fixdt(1, 16)  ParameterScaling=2^0  OutDataType=fixdt(1, 16)  OutScaling=2^0
  Math Function : Math  DisableCoverage=on  Operator=rem  OutDataType=fixdt(1, 16)  OutScaling=2^0  SaturateOnIntegerOverflow=on
  saw : Outport
  wires:
  Constant/1 -> Math Function/2, Divide/2
  Clock/1 -> Math Function/1
  Math Function/1 -> Divide/1
  Divide/1 -> Gain/1
  Gain/1 -> saw/1
